simulink model "CommunicationSystemsLab10Task2"  (R2015a)
settings: Solver=ode45  StartTime=0.0  StopTime=10.0  RelTol=1e-3
settings Model: Creator=Quswar Mahmood Abid  LastModifiedBy=Quswar Mahmood Abid

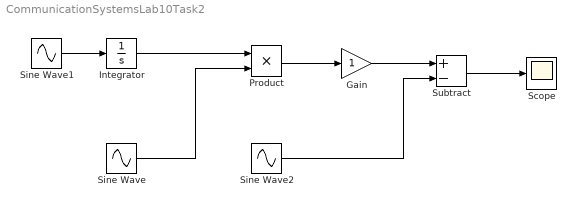
== system CommunicationSystemsLab10Task2 ==
  Gain : Gain
  Integrator : Integrator
  Product : Product
  Scope : Scope
  Sine Wave : Sin  SampleTime=0
  Sine Wave1 : Sin  Frequency=10000  SampleTime=0
  Sine Wave2 : Sin  SampleTime=0
  Subtract : Sum  Inputs=+-
  wires:
  Sine Wave/1 -> Product/2
  Integrator/1 -> Product/1
  Product/1 -> Gain/1
  Subtract/1 -> Scope/1
  Gain/1 -> Subtract/1
  Sine Wave1/1 -> Integrator/1
  Sine Wave2/1 -> Subtract/2
